simulink model "nonlinear_system"  (R2024b)
settings: Solver=VariableStepAuto  StartTime=0.0  StopTime=Tf  RelTol=1e-3
values from neighbouring files (symbols this model uses):
  g = 9.81    [script_rotating_disk.m]
  J = 1    [script_rotating_disk.m]
  m = 1    [script_rotating_disk.m]
  theta0 = 20    [script_rotating_disk.m]
  x0 = [si dotsi wi]    [script_rotating_disk.m]
settings Model: Creator=martinhaugen  LastModifiedBy=martinhaugen

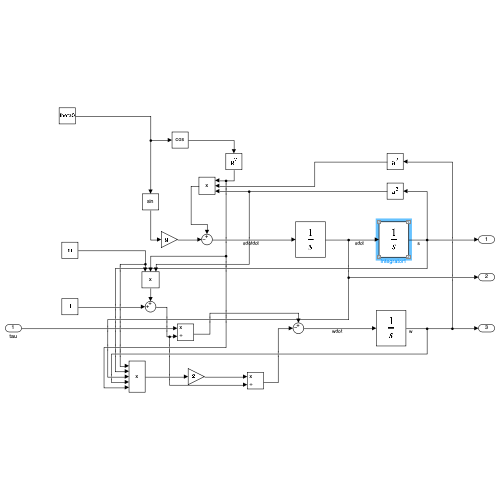
[thumbnail: Simulink's stored preview of the top-level diagram]
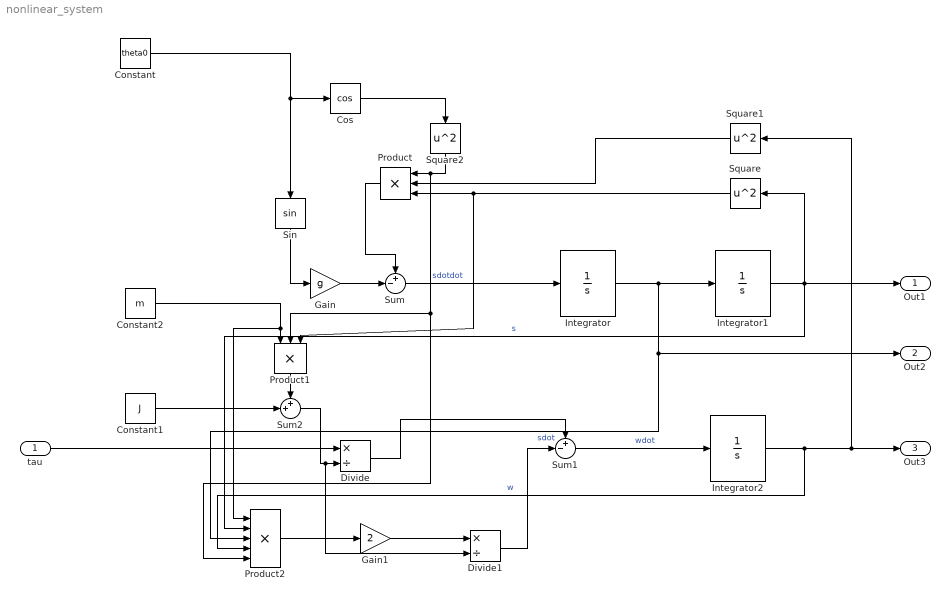
== system nonlinear_system ==
  tau : Inport
  Constant : Constant  Value=theta0
  Constant1 : Constant  Value=J
  Constant2 : Constant  Value=m
  Cos : Trigonometry  Operator=cos
  Divide : Product  Inputs=*/
  Divide1 : Product  Inputs=*/
  Gain : Gain  Gain=g
  Gain1 : Gain  Gain=2
  Integrator : Integrator  InitialCondition=x0(2)
  Integrator1 : Integrator  InitialCondition=x0(1)
  Integrator2 : Integrator  InitialCondition=x0(3)
  Product : Product  Inputs=3
  Product1 : Product  Inputs=3
  Product2 : Product  Inputs=5
  Sin : Trigonometry
  Square : Math  Operator=square
  Square1 : Math  Operator=square
  Square2 : Math  Operator=square
  Sum : Sum  Inputs=+-|
  Sum1 : Sum  Inputs=+-|
  Sum2 : Sum  Inputs=++|
  Out1 : Outport
  Out2 : Outport  Port=2
  Out3 : Outport  Port=3
  wires:
  Sum/1 -> Integrator/1  "sdotdot"
  Integrator/1 -> Out2/1, Product2/3, Integrator1/1  "sdot"
  Integrator1/1 -> Product2/2, Out1/1, Square/1  "s"
  Sum1/1 -> Integrator2/1  "wdot"
  Integrator2/1 -> Product2/4, Out3/1, Square1/1  "w"
  Product/1 -> Sum/1
  Constant/1 -> Sin/1, Cos/1
  Cos/1 -> Square2/1
  Square2/1 -> Product1/2, Product2/5, Product/1
  Square1/1 -> Product/2
  Square/1 -> Product1/3, Product/3
  Sin/1 -> Gain/1
  Gain/1 -> Sum/2
  tau/1 -> Divide/1
  Divide/1 -> Sum1/1
  Constant1/1 -> Sum2/2
  Product1/1 -> Sum2/1
  Constant2/1 -> Product2/1, Product1/1
  Sum2/1 -> Divide1/2, Divide/2
  Divide1/1 -> Sum1/2
  Gain1/1 -> Divide1/1
  Product2/1 -> Gain1/1
